simulink model "rock_paper_scissors"  (R2021a)
settings: Solver=VariableStepAuto  StartTime=0.0  StopTime=inf  RelTol=1e-3
libraries: vrlib x1
settings Model: Creator=kbhar  LastModifiedBy=kbhar

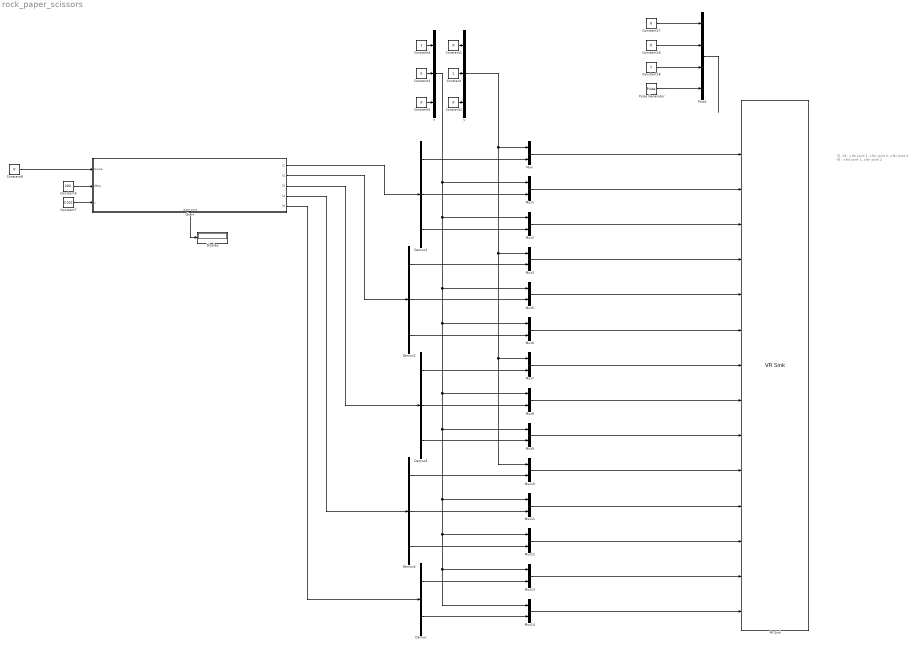
== system rock_paper_scissors ==
  note: f1 - f4 : y for joint 1, x for joint 2, x for joint 3
      | f5 : x for joint 1, x for joint 2
  Chart : Stateflow chart  TreatAsAtomicUnit=on
      settings: PortSchema="{\"entries\":[{\"content\":{\"sides\":[{\"content\":{\"connectorIds\":[\"In1\",\"In2\",\"In3\"]},\"type\":\"ConnectorPlacement.EquallySpacedRectSide\",\"uuid\":\"4f0c7b3f-89a5-412d-9997-362734ab353d\"},{\"content\":{\"connectorIds\":[\"Out1\",\"Out2\",\"Out3\",\"Out4\",\"Out5\"],\"side\":\"RIGHT\"},\"type\":\"ConnectorPlacement.EquallySpacedRectSide\",\"uuid\":\"1b9ed4a9-8110-455e-a273-14ccb808f4d5\"},{\"content\":{\"connectorIds\":[],\"side\":\"TOP\"},\"type\":\"ConnectorPlacement.EquallySpacedRectSide\",\"uuid\":\"910bd171-52a2-4250-814e-2d79bc985340\"},{\"content\":{\"connectorIds\":[\"Out6\"],\"side\":\"BOTTOM\"},\"type\":\"ConnectorPlacement.EquallySpacedRectSide\",\"uuid\":\"18cd32ff-89aa-47da-893b-8a990fce90ad\"}]},\"type\":\"ConnectorPlacement.EquallySpacedConnector\",\"uuid\":\"baa157e6-4c19-4506-8586-4b17a33aaba9\"}],\"packageUris\":[\"http://schema.mathworks.com/mf0/Connector/R2020b\"],\"version\":\"1.0\"}"
  Constant : Constant
  Constant{1..3,5,8,16..17} (7 alike) : Constant  Value=0
  Constant18 : Constant
  Constant4 : Constant
  Constant6 : Constant  Value=200
  Constant7 : Constant  Value=0.002
  Demux : Demux  Outputs=2
  Demux{1..4} (4 alike) : Demux  Outputs=3
  Display : Display
  Mux{,1..3,5..14} (14 alike) : Mux  Inputs=2
  Mux4 : Mux
  Pulse Generator : DiscretePulseGenerator  PulseType=Time based  Amplitude=pi/15  Period=20  PulseWidth=50
  VR Sink : vrlib/VR Sink  InstantiateOnLoad=on  SampleTime=0.1  ViewEnable=on  RemoteChange=off  RemoteView=off  FieldsWritten=palm.rotation.4.1.1.double#f1joint1.rotation.4.1.1.double#f1joint2.rotation.4.1.1.double#f1joint3.rotation.4.1.1.double#f2joint1.rotation.4.1.1.double#f2joint2.rotation.4.1.1.double#f2joint3.rotation.4.1.1.double#f3joint1.rotation.4.1.1.double#f3joint2.rotation.4.1.1.double#f3joint3.rotation.4.1.1.double#f4joint1.rotation.4.1.1.double#f4joint2.rotation.4.1.1.double#f4joint3.rotation.4.1.1.double#f5joint1.rotation.4.1.1.double#f5joint2.rotation.4.1.1.double  WorldFileName=rock_paper_scissors.wrl  AutoView=off  VideoDimensions=[]  AllowVariableSize=off
  x : Mux  Inputs=3
  y : Mux  Inputs=3
  wires:
  Constant/1 -> y/2
  Constant1/1 -> y/1
  Constant2/1 -> y/3
  Pulse Generator/1 -> Mux4/4
  Constant18/1 -> Mux4/3
  Constant17/1 -> Mux4/1
  Constant16/1 -> Mux4/2
  Mux4/1 -> ?
  Mux/1 -> VR Sink/2
  Mux1/1 -> VR Sink/3
  Mux3/1 -> VR Sink/5
  Mux2/1 -> VR Sink/4
  Mux7/1 -> VR Sink/8
  Mux8/1 -> VR Sink/9
  Mux6/1 -> VR Sink/7
  Mux5/1 -> VR Sink/6
  Mux11/1 -> VR Sink/12
  Mux12/1 -> VR Sink/13
  Mux14/1 -> VR Sink/15
  Mux13/1 -> VR Sink/14
  Mux9/1 -> VR Sink/10
  Mux10/1 -> VR Sink/11
  Constant5/1 -> x/3
  Constant4/1 -> x/1
  Constant3/1 -> x/2
  y/1 -> Mux10/1, Mux7/1, Mux3/1, Mux/1
  x/1 -> Mux5/1, Mux6/1, Mux8/1, Mux9/1, Mux11/1, Mux12/1, Mux13/1, Mux14/1, Mux2/1, Mux1/1
  Chart/5(f5) -> Demux/1
  Demux/2 -> Mux14/2
  Demux/1 -> Mux13/2
  Demux1/1 -> Mux/2
  Demux1/2 -> Mux1/2
  Demux1/3 -> Mux2/2
  Demux2/3 -> Mux6/2
  Demux2/2 -> Mux5/2
  Demux2/1 -> Mux3/2
  Demux4/1 -> Mux10/2
  Demux4/2 -> Mux11/2
  Demux4/3 -> Mux12/2
  Demux3/3 -> Mux9/2
  Demux3/2 -> Mux8/2
  Demux3/1 -> Mux7/2
  Chart/1(f1) -> Demux1/1
  Chart/2(f2) -> Demux2/1
  Chart/3(f3) -> Demux3/1
  Chart/4(f4) -> Demux4/1
  Constant7/1 -> Chart/3(x)
  Chart/6(reset_time) -> Display/1
  Constant6/1 -> Chart/2(delay)
  Constant8/1 -> Chart/1(choice)

== stateflow chart rock_paper_scissors/Chart ==
  state rock_state1
    f1 = f1 + x; f2 = f2 + x; f3 = f3 + x; f4 = f4 + x; f5 = f5 + x;
  state rock_state2
    f1 = [pi/2 pi/2 pi/2]; f2 = [pi/2 pi/2 pi/2]; f3 = [pi/2 pi/2 pi/2]; f4 = [pi/2 pi/2 pi/2]; f5 = [pi/2 pi/2];
  state rock_state3
    f1 = f1 - x; f2 = f2 - x; f3 = f3 - x; f4 = f4 - x; f5 = f5 - x; reset_time = 1;
  state rock_pause_state
    f1 = [0 0 0]; f2 = [0 0 0]; f3 = [0 0 0]; f4 = [0 0 0]; f5 = [0 0];
  state scissor_state1
    f3 = f3 + x; f4 = f4 + x; f5 = f5 + x;
  state scissor_state2
    f3 = [pi/2 pi/2 pi/2]; f4 = [pi/2 pi/2 pi/2]; f5 = [pi/2 pi/2];
  state scissor_state3
    f3 = f3 - x; f4 = f4 - x; f5 = f5 - x; reset_time = 1;
  state startstate
    f1 = [0 0 0]; f2 = [0 0 0]; f3 = [0 0 0]; f4 = [0 0 0]; f5 = [0 0]; reset_time = 0;
  state scissor_pause_state
    f1 = [0 0 0]; f2 = [0 0 0]; f3 = [0 0 0]; f4 = [0 0 0]; f5 = [0 0];
  state paper_state1
  state paper_state2
  state paper_state3
    reset_time = 1;
  state paper_pause_state
    f1 = [0 0 0]; f2 = [0 0 0]; f3 = [0 0 0]; f4 = [0 0 0]; f5 = [0 0];
  rock_state2 -> rock_state3 : [delay >= 150]
  rock_pause_state -> rock_state1 : [delay >= 50]
  rock_state1 -> rock_state2 : [f1(1) >= pi/2 - x]
  rock_state3 -> startstate : [f1(1) <=x]
  startstate -> rock_pause_state [order 1] : [choice == 0]
  (default) -> startstate
  startstate -> scissor_pause_state [order 2] : [choice == 1]
  scissor_pause_state -> scissor_state1 : [delay >= 50]
  scissor_state2 -> scissor_state3 : [delay >= 150]
  scissor_state1 -> scissor_state2 : [f3(1) >= pi/2 - x]
  scissor_state3 -> startstate : [f3(1) <=x]
  paper_state3 -> startstate : [f1(1) <=x]
  startstate -> paper_pause_state [order 3] : [choice == 2]
  paper_state2 -> paper_state3 : [delay >= 150]
  paper_state1 -> paper_state2 : [f1(1) >= 0]
  paper_pause_state -> paper_state1 : [delay >= 50]
  data: f1 output; f2 output; f3 output; f4 output; f5 output; choice input; delay input; x input; reset_time output
